simulink model "vrbounce"  (Simulink 6.0)
settings: Solver=ode45  SolverMode=SingleTasking  StartTime=0.0  StopTime=Inf  FixedStep=0.02  RelTol=1e-3
libraries: vrlib x2
settings Model: CovMetricSettings=d  Creator=Straka  LastModifiedBy=Houska  ExtModeTrigDuration=500
settings DataIOCC: LimitDataPoints=off  SaveOutput=off  SaveTime=off  SignalLoggingName=logsOut
settings OptimizationCC: BlockReduction=off  BooleanDataType=off
settings DebuggingCC: CheckExecutionContextPreStartOutputMsg=on  CheckExecutionContextRuntimeOutputMsg=on  SolverPrmCheckMsg=none
settings HardwareCC: TargetUnknown=on
settings ModelReferenceCC: UpdateModelReferenceTargets=IfOutOfDate
settings GRTTargetCC: LifeSpan=inf
settings SFSimCC: SFSimApplyToAllLibs=on  SFSimBuildMode=Incremental

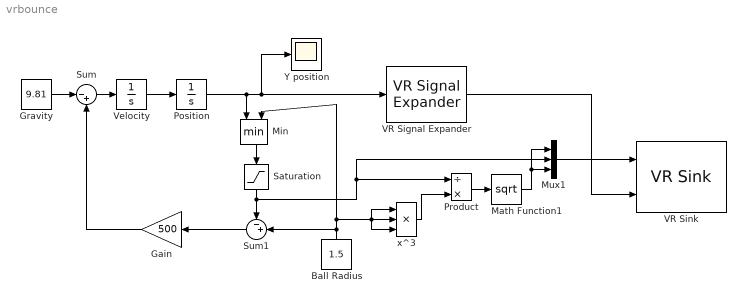
== system vrbounce ==
  Ball Radius : Constant  Orientation=up  Value=1.5
  Gain : Gain  Orientation=left  Gain=500  SaturateOnIntegerOverflow=on
  Gravity : Constant  Value=9.81
  Math Function1 : Math  Operator=sqrt  SaturateOnIntegerOverflow=on
  Min : MinMax  Orientation=down  Inputs=2  ZeroCross=off  SaturateOnIntegerOverflow=on  InputSameDT=on
  Mux1 : Mux  Inputs=3
  Position : Integrator  InitialCondition=20  UpperSaturationLimit=Inf  LowerSaturationLimit=-Inf  ZeroCross=off
  Product : Product  Inputs=/*  SaturateOnIntegerOverflow=on  InputSameDT=on
  Saturation : Saturate  Orientation=down  UpperLimit=Inf  LowerLimit=0  ZeroCross=off
  Sum : Sum  Inputs=|-+  SaturateOnIntegerOverflow=on  InputSameDT=on
  Sum1 : Sum  Orientation=left  Inputs=-+|  SaturateOnIntegerOverflow=on  InputSameDT=on
  VR Signal Expander : vrlib/VR Signal Expander  outwidth=3  outidx=2
  VR Sink : vrlib/VR Sink  SampleTime=0.02  ViewEnable=on  RemoteChange=off  RemoteView=off  FieldsWritten=Ball.scale.3.1.double#Ball.translation.3.1.double  WorldFileName=vrbounce.wrl  AutoView=on
  Velocity : Integrator  UpperSaturationLimit=Inf  LowerSaturationLimit=-Inf  ZeroCross=off
  Y position : Scope
      settings: TimeRange=10  YMin=0  YMax=20
  x^3 : Product  Inputs=3  SaturateOnIntegerOverflow=on  InputSameDT=on
  wires:
  Velocity/1 -> Position/1
  Mux1/1 -> VR Sink/1
  VR Signal Expander/1 -> VR Sink/2
  Sum/1 -> Velocity/1
  Gravity/1 -> Sum/1
  Position/1 -> Y position/1, VR Signal Expander/1, Min/1
  Gain/1 -> Sum/2
  Min/1 -> Saturation/1
  Sum1/1 -> Gain/1
  Saturation/1 -> Sum1/1, Mux1/2, Product/1
  Product/1 -> Math Function1/1
  x^3/1 -> Product/2
  Math Function1/1 -> Mux1/1, Mux1/3
  Ball Radius/1 -> Sum1/2, Min/2, x^3/2, x^3/1, x^3/3
